simulink model "Loop_TestModel"  (R2014a)
settings: Solver=ode45  StartTime=0.0  StopTime=10.0  RelTol=1e-3
libraries: rocket_drag_library x1, rocket_isa_model_library x1, rocket_vertical_flight_library x1
settings Model: Creator=scorpii  LastModifiedBy=scorpii

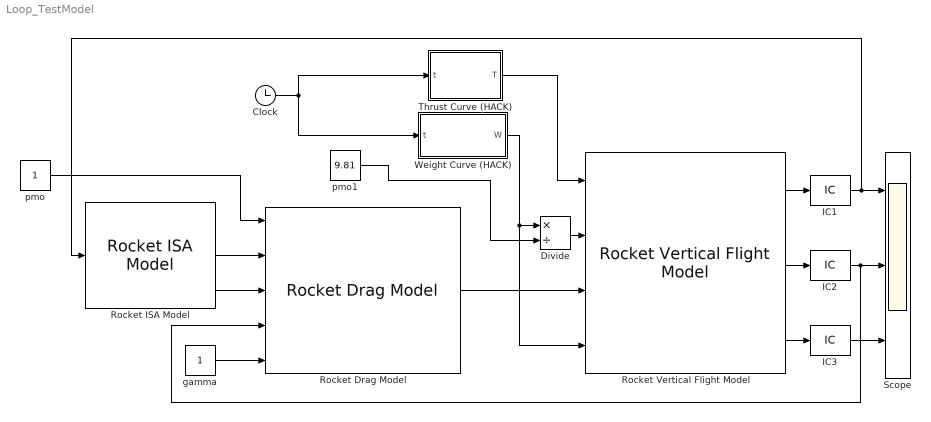
== system Loop_TestModel ==
  Clock : Clock
  Divide : Product  Inputs=*/
  IC1 : InitialCondition
  IC2 : InitialCondition  Value=0
  IC3 : InitialCondition  Value=0
  Rocket Drag Model : rocket_drag_library/Rocket Drag Model
      link override Drag Force/BasicDrag: MATLABFcn=BasicDrag
      link override Skin Friction Drag Coefficient/Actual Reynolds Number/Reynolds Number (Actual): MATLABFcn=ReynoldsNumberActual
  Rocket ISA Model : rocket_isa_model_library/Rocket ISA Model
  Rocket Vertical Flight Model : rocket_vertical_flight_library/Rocket Vertical Flight Model
  Scope : Scope  NumInputPorts=3
      settings: YMin=-5~-5~-5  YMax=5~5~5
  Thrust Curve (HACK) : MATLAB Function  TreatAsAtomicUnit=on
  Weight Curve (HACK) : MATLAB Function  TreatAsAtomicUnit=on
  gamma : Constant
  pmo : Constant
  pmo1 : Constant  Value=9.81
  wires:
  Rocket ISA Model/2 -> Rocket Drag Model/2
  Rocket ISA Model/3 -> Rocket Drag Model/3
  gamma/1 -> Rocket Drag Model/5
  Rocket Vertical Flight Model/2 -> IC2/1
  pmo/1 -> Rocket Drag Model/1
  Rocket Vertical Flight Model/1 -> IC1/1
  Rocket Drag Model/1 -> Rocket Vertical Flight Model/3
  Thrust Curve (HACK)/1(T) -> Rocket Vertical Flight Model/1
  Weight Curve (HACK)/1(W) -> Divide/1, Rocket Vertical Flight Model/4
  Clock/1 -> Thrust Curve (HACK)/1(t), Weight Curve (HACK)/1(t)
  Divide/1 -> Rocket Vertical Flight Model/2
  pmo1/1 -> Divide/2
  Rocket Vertical Flight Model/3 -> IC3/1
  IC3/1 -> Scope/3
  IC2/1 -> Rocket Drag Model/4, Scope/2
  IC1/1 -> Rocket ISA Model/1, Scope/1

== matlab function Loop_TestModel/Weight Curve (HACK) ==
  data: W output; t input
function W = weight_hack(t)

if t<0.47775
    W=(-36625*t^4+32622*t^3-9361.4*t^2-112.87*t+21203)/1000*9.80665 
elseif t<4.0777
    W=(60.388*t^2-1213.3*t+21312)/1000*9.80665 
elseif t<4.5777
    W=(-144.73*t+18078)/1000*9.80665 
else
    W=17422/1000*9.80665 
end

end

== matlab function Loop_TestModel/Thrust Curve (HACK) ==
  data: t input; T output
function T = thrust_hack(t)
    if t<0.08
    T=4000000*t^3-462933*t^2+41915*t+209.66;
    elseif t<0.15935
    T=-4701*t+2748.7;
    elseif t<0.21276 
    T=-1133.2*t+2223.6 ;
    elseif t<0.32775
    T=787.15*t+1850.2;
    elseif t<0.57775
    T=-754.4*t+2339.9;
    elseif t<0.72775
    T=-251*t+2070.7 ;
    elseif t<1.7277
    T=-70.147*t+1947.4;
    elseif t<3.3777
    T=-31.421*t^2-9.1503*t+1930.8;
    elseif t<3.9777
    T=3656.6*t^3-39167*t^2+137806*t-158018;
    elseif t<4.5277
    T=-1051.8*t+4709.4;
    else
    T=0;
end
